simulink model "Bool"  (R2018a)
settings: Solver=VariableStepAuto  StartTime=0.0  StopTime=inf  RelTol=1e-3
libraries: opclib x3
settings Model: Creator=gabrielgbm  LastModifiedBy=gabrielgbm

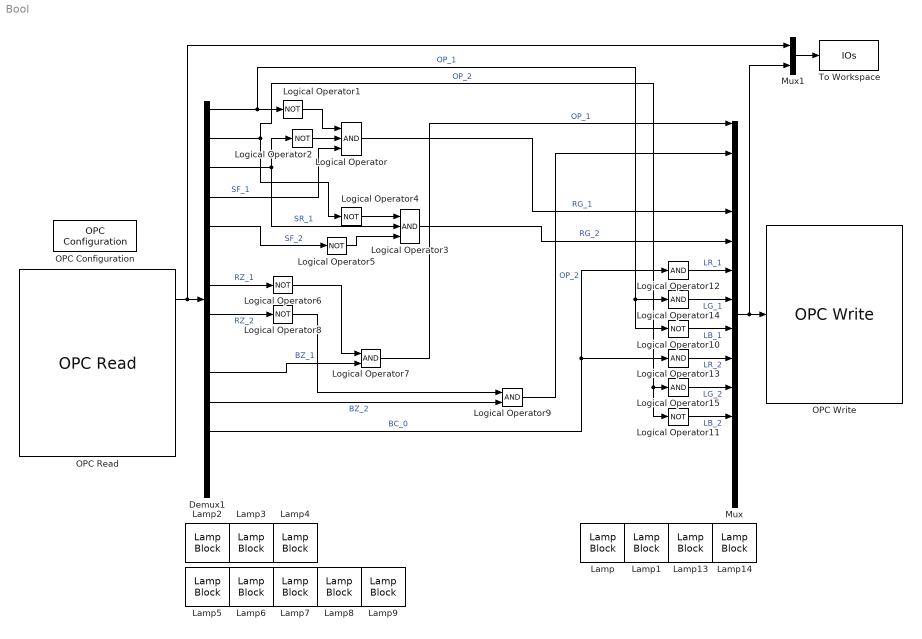
== system Bool ==
  Demux1 : Demux  Outputs=14
  Lamp : LampBlock  WebBlockId=47
  Lamp1 : LampBlock  WebBlockId=48
  Lamp13 : LampBlock  WebBlockId=67
  Lamp14 : LampBlock  WebBlockId=68
  Lamp2 : LampBlock  WebBlockId=53
  Lamp3 : LampBlock  WebBlockId=54
  Lamp4 : LampBlock  WebBlockId=55
  Lamp5 : LampBlock  WebBlockId=59
  Lamp6 : LampBlock  WebBlockId=60
  Lamp7 : LampBlock  WebBlockId=61
  Lamp8 : LampBlock  WebBlockId=62
  Lamp9 : LampBlock  WebBlockId=63
  Logical Operator : Logic  Inputs=3  IconShape=distinctive  AllPortsSameDT=off  OutDataTypeStr=boolean
  Logical Operator{1..2,4..6,8,10..11} (8 alike) : Logic  Operator=NOT  IconShape=distinctive  AllPortsSameDT=off  OutDataTypeStr=boolean
  Logical Operator{12..15} (4 alike) : Logic  Inputs=1  IconShape=distinctive  AllPortsSameDT=off  OutDataTypeStr=boolean
  Logical Operator3 : Logic  Inputs=3  IconShape=distinctive  AllPortsSameDT=off  OutDataTypeStr=boolean
  Logical Operator7 : Logic  IconShape=distinctive  AllPortsSameDT=off  OutDataTypeStr=boolean
  Logical Operator9 : Logic  IconShape=distinctive  AllPortsSameDT=off  OutDataTypeStr=boolean
  Mux : Mux  Inputs=14
  Mux1 : Mux  Inputs=2
  OPC Configuration : opclib/OPC Configuration  opcServers=localhost/Matrikon.OPC.GDA.1/10  errMissingItems=Error  errReadWrite=Warn  errShutdown=Error  errRTViolation=Warn  rtEnable=on  speedup=1  showLatency=off  beingUsed=on
      settings: SourceProductName=OPC Toolbox  SourceProductBaseCode=OT
  OPC Read : opclib/OPC Read  serverHost=localhost  serverID=Matrikon.OPC.GDA.1  itemIDs=Sinais.PLC_OP_1, Sinais.PLC_OP_2, Sinais.PLC_SR_1, Sinais.PLC_SF_1, Sinais.PLC_SF_2, Sinais.PLC_RZ_0, Sinais.PLC_RZ_1, Sinais.PLC_RZ_2, Sinais.PLC_RI_1, Sinais.PLC_BZ_1, Sinais.PLC_BZ_2, Sinais.PLC_BC_0, Sinais.PLC_BC_1, Sinais.PLC_BC_2  readMode=Synchronous (cache)  dataType=logical  updateRate=0.5  showQual=on  showTS=on  tsMode=Seconds since start
      settings: SourceProductName=OPC Toolbox  SourceProductBaseCode=OT
  OPC Write : opclib/OPC Write  serverHost=localhost  serverID=Matrikon.OPC.GDA.1  itemIDs=Sinais.PLC_OP_1, Sinais.PLC_OP_2, Sinais.PLC_RG_0, Sinais.PLC_RG_1, Sinais.PLC_RG_2, Sinais.PLC_LR_1, Sinais.PLC_LG_1, Sinais.PLC_LB_1, Sinais.PLC_LR_2, Sinais.PLC_LG_2, Sinais.PLC_LB_2, Sinais.PLC_RO_0, Sinais.PLC_RO_1, Sinais.PLC_RO_2  writeMode=Synchronous  updateRate=0
      settings: SourceProductName=OPC Toolbox  SourceProductBaseCode=OT
  To Workspace : ToWorkspace  VariableName=IOs  SampleTime=1
  wires:
  Mux/1 -> Mux1/2, OPC Write/1
  Demux1/1 -> Logical Operator14/1, Logical Operator10/1, Logical Operator1/1  "OP_1"
  Logical Operator1/1 -> Logical Operator/1
  Logical Operator2/1 -> Logical Operator/2
  Demux1/4 -> Logical Operator/3  "SF_1"
  Logical Operator/1 -> Mux/4  "RG_1"
  Demux1/3 -> Logical Operator3/2, Logical Operator2/1  "SR_1"
  Logical Operator4/1 -> Logical Operator3/1
  Logical Operator3/1 -> Mux/5  "RG_2"
  Demux1/2 -> Logical Operator4/1, Logical Operator15/1, Logical Operator11/1  "OP_2"
  Logical Operator5/1 -> Logical Operator3/3
  Demux1/5 -> Logical Operator5/1  "SF_2"
  Demux1/7 -> Logical Operator6/1  "RZ_1"
  Logical Operator7/1 -> Mux/1  "OP_1"
  Demux1/8 -> Logical Operator8/1  "RZ_2"
  OPC Read/1 -> Mux1/1, Demux1/1
  Logical Operator10/1 -> Mux/8  "LB_1"
  Logical Operator11/1 -> Mux/11  "LB_2"
  Logical Operator9/1 -> Mux/2  "OP_2"
  Logical Operator12/1 -> Mux/6  "LR_1"
  Logical Operator13/1 -> Mux/9  "LR_2"
  Demux1/12 -> Logical Operator13/1, Logical Operator12/1  "BC_0"
  Logical Operator14/1 -> Mux/7  "LG_1"
  Logical Operator15/1 -> Mux/10  "LG_2"
  Demux1/10 -> Logical Operator7/2  "BZ_1"
  Demux1/11 -> Logical Operator9/2  "BZ_2"
  Mux1/1 -> To Workspace/1
  Logical Operator6/1 -> Logical Operator7/1
  Logical Operator8/1 -> Logical Operator9/1
